simulink model "W04_1_sensor_rates"  (R2024b)
settings: Solver=FixedStepDiscrete  StartTime=0.0  StopTime=T_end  FixedStep=Ts  RelTol=1e-3
values from neighbouring files (symbols this model uses):
  Ts = 0.05    [W04_heading_sign.m]    (also in W04_offline_run.m = evalin('base','Ts'); W04_setup.m = 0.005)
libraries: ros2lib x3
settings Model: Creator=admin  LastModifiedBy=admin

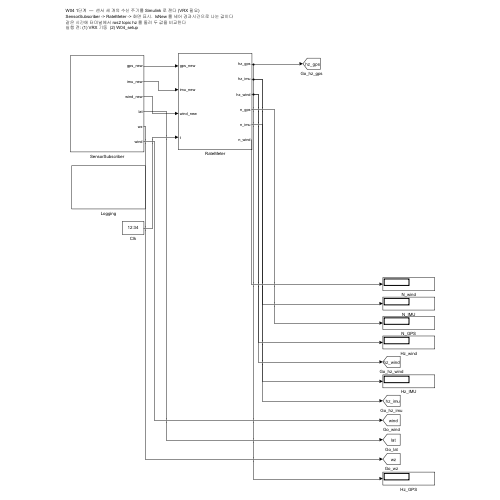
[thumbnail: Simulink's stored preview of the top-level diagram]
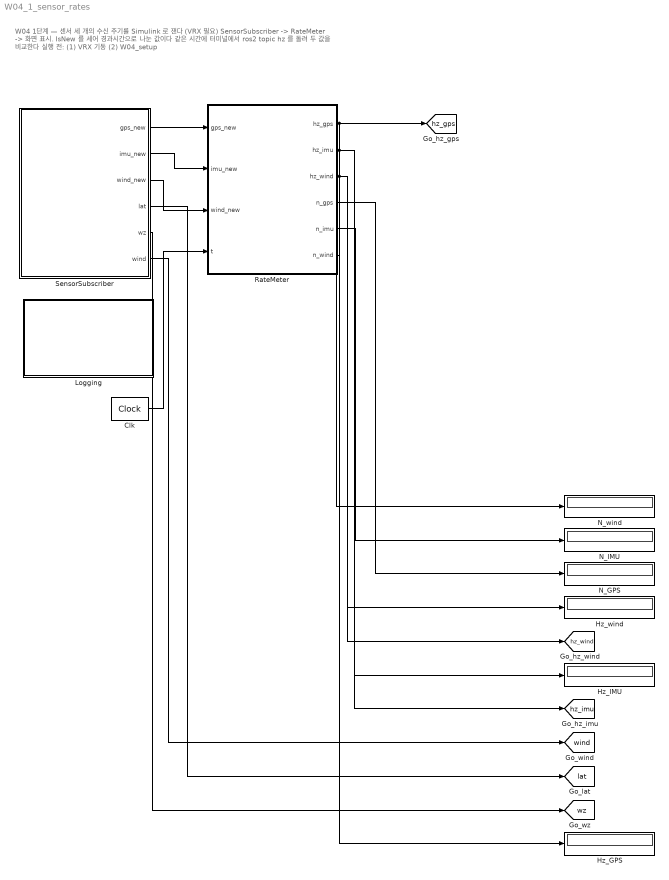
== system W04_1_sensor_rates ==
  note: W04 1단계  —  센서 세 개의 수신 주기를 Simulink 로 잰다 (VRX 필요)
      | SensorSubscriber -> RateMeter -> 화면 표시.  IsNew 를 세어 경과시간으로 나눈 값이다
      | 같은 시간에 터미널에서 ros2 topic hz 를 돌려 두 값을 비교한다
      | 실행 전: (1) VRX 기동  (2) W04_setup
  Clk : DigitalClock  SampleTime=Ts
  Hz_GPS : Display
  Hz_IMU : Display
  Hz_wind : Display
  Logging : Subsystem
  N_GPS : Display
  N_IMU : Display
  N_wind : Display
  RateMeter : Subsystem
  SensorSubscriber : Subsystem
  tag scope: hz_gps=global, hz_imu=global, hz_wind=global, lat=global, wind=global, wz=global
  wires:
  SensorSubscriber/1(gps_new) -> RateMeter/1(gps_new)
  SensorSubscriber/2(imu_new) -> RateMeter/2(imu_new)
  SensorSubscriber/3(wind_new) -> RateMeter/3(wind_new)
  Clk/1 -> RateMeter/4(t)
  RateMeter/6(n_wind) -> N_wind/1
  RateMeter/5(n_imu) -> N_IMU/1
  RateMeter/4(n_gps) -> N_GPS/1
  SensorSubscriber/6(wind) -> [wind]
  SensorSubscriber/4(lat) -> [lat]
  SensorSubscriber/5(wz) -> [wz]
  RateMeter/1(hz_gps) -> [hz_gps], Hz_GPS/1
  RateMeter/3(hz_wind) -> [hz_wind], Hz_wind/1
  RateMeter/2(hz_imu) -> [hz_imu], Hz_IMU/1

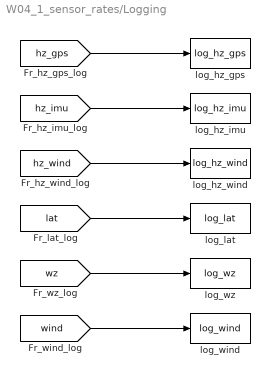
== system W04_1_sensor_rates/Logging ==
  log_hz_gps : ToWorkspace  VariableName=log_hz_gps  SaveFormat=Timeseries  SampleTime=Ts
  log_hz_imu : ToWorkspace  VariableName=log_hz_imu  SaveFormat=Timeseries  SampleTime=Ts
  log_hz_wind : ToWorkspace  VariableName=log_hz_wind  SaveFormat=Timeseries  SampleTime=Ts
  log_lat : ToWorkspace  VariableName=log_lat  SaveFormat=Timeseries  SampleTime=Ts
  log_wind : ToWorkspace  VariableName=log_wind  SaveFormat=Timeseries  SampleTime=Ts
  log_wz : ToWorkspace  VariableName=log_wz  SaveFormat=Timeseries  SampleTime=Ts
  wires:
  [hz_gps] -> log_hz_gps/1
  [hz_imu] -> log_hz_imu/1
  [hz_wind] -> log_hz_wind/1
  [lat] -> log_lat/1
  [wz] -> log_wz/1
  [wind] -> log_wind/1

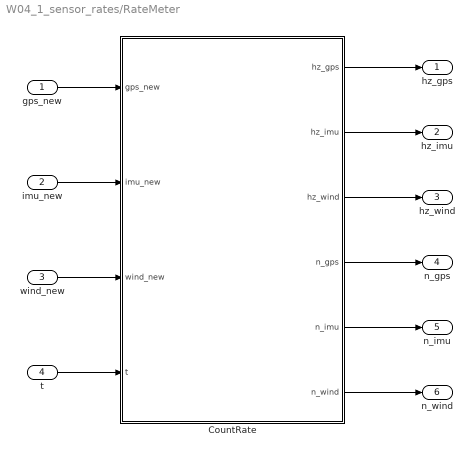
== system W04_1_sensor_rates/RateMeter ==
  gps_new : Inport
  imu_new : Inport  Port=2
  wind_new : Inport  Port=3
  t : Inport  Port=4
  CountRate : MATLAB Function  TreatAsAtomicUnit=on
  hz_gps : Outport
  hz_imu : Outport  Port=2
  hz_wind : Outport  Port=3
  n_gps : Outport  Port=4
  n_imu : Outport  Port=5
  n_wind : Outport  Port=6
  wires:
  CountRate/3(hz_wind) -> hz_wind/1
  gps_new/1 -> CountRate/1(gps_new)
  t/1 -> CountRate/4(t)
  imu_new/1 -> CountRate/2(imu_new)
  wind_new/1 -> CountRate/3(wind_new)
  CountRate/2(hz_imu) -> hz_imu/1
  CountRate/1(hz_gps) -> hz_gps/1
  CountRate/4(n_gps) -> n_gps/1
  CountRate/5(n_imu) -> n_imu/1
  CountRate/6(n_wind) -> n_wind/1

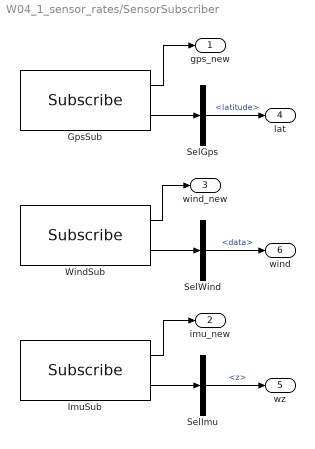
== system W04_1_sensor_rates/SensorSubscriber ==
  GpsSub : ros2lib/Subscribe  topicSource=Specify your own  topic=/wamv/sensors/gps/gps/fix  messageType=sensor_msgs/NavSatFix  sampleTime=Ts  QOSHistory=Keep last  QOSDepth=1  QOSReliability=Reliable  QOSDurability=Volatile  QOSDeadline=Inf  QOSLifespan=Inf  QOSLiveliness=Automatic  QOSLeaseDuration=Inf  QOSAvoidROSNamespaceConventions=off
  ImuSub : ros2lib/Subscribe  topicSource=Specify your own  topic=/wamv/sensors/imu/imu/data  messageType=sensor_msgs/Imu  sampleTime=Ts  QOSHistory=Keep last  QOSDepth=1  QOSReliability=Reliable  QOSDurability=Volatile  QOSDeadline=Inf  QOSLifespan=Inf  QOSLiveliness=Automatic  QOSLeaseDuration=Inf  QOSAvoidROSNamespaceConventions=off
  SelGps : BusSelector  OutputSignals=latitude
  SelImu : BusSelector  OutputSignals=angular_velocity.z
  SelWind : BusSelector  OutputSignals=data
  WindSub : ros2lib/Subscribe  topicSource=Specify your own  topic=/vrx/debug/wind/speed  messageType=std_msgs/Float32  sampleTime=Ts  QOSHistory=Keep last  QOSDepth=1  QOSReliability=Reliable  QOSDurability=Volatile  QOSDeadline=Inf  QOSLifespan=Inf  QOSLiveliness=Automatic  QOSLeaseDuration=Inf  QOSAvoidROSNamespaceConventions=off
  gps_new : Outport
  imu_new : Outport  Port=2
  wind_new : Outport  Port=3
  lat : Outport  Port=4
  wz : Outport  Port=5
  wind : Outport  Port=6
  wires:
  SelGps/1 -> lat/1  "<latitude>"
  GpsSub/1 -> gps_new/1
  WindSub/2 -> SelWind/1
  WindSub/1 -> wind_new/1
  ImuSub/2 -> SelImu/1
  SelWind/1 -> wind/1  "<data>"
  GpsSub/2 -> SelGps/1
  ImuSub/1 -> imu_new/1
  SelImu/1 -> wz/1  "<z>"

== matlab function W04_1_sensor_rates/RateMeter/CountRate ==
  data: gps_new input; hz_gps output; imu_new input; wind_new input; t input; hz_imu output; hz_wind output; n_gps output; n_imu output; n_wind output
function [hz_gps, hz_imu, hz_wind, n_gps, n_imu, n_wind] = CountRate(gps_new, imu_new, wind_new, t)
%#codegen
% Count how many messages arrived and divide by elapsed time.
% This is what `ros2 topic hz` does, on the same wall clock.
persistent cg ci cw
if isempty(cg), cg = 0; ci = 0; cw = 0; end
if gps_new,  cg = cg + 1; end
if imu_new,  ci = ci + 1; end
if wind_new, cw = cw + 1; end

n_gps = cg;  n_imu = ci;  n_wind = cw;
if t > 0
    hz_gps = cg/t;  hz_imu = ci/t;  hz_wind = cw/t;
else
    hz_gps = 0;     hz_imu = 0;     hz_wind = 0;
end
